simulink model "ProcessFlowRateModel_symbiotic_2014APR18"  (Simulink 7.9)
settings: Solver=VariableStepDiscrete  StartTime=0.0  StopTime=10000  RelTol=1e-3
libraries: simeventslib x9
(part 1 of 2)
settings Model: Creator=tsprock3  LastModifiedBy=tsprock3
settings DebuggingCC: SimStateOlderReleaseMsg=warning

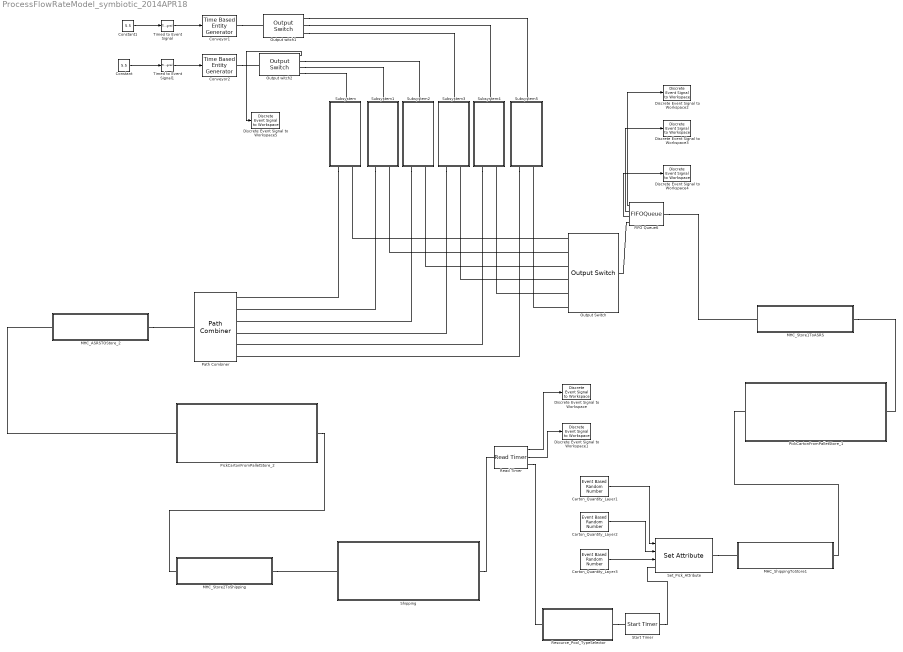
== system ProcessFlowRateModel_symbiotic_2014APR18 ==
  Carton_Quantity_Layer1 : EventBasedRandomNumber  Distribution=Discrete uniform  minUnid=17  maxUnid=23  numValueUnid=7  valueVecDisc=[1 2 3]  probVecDisc=[0.5 0.35 0.15]  Seed=35621
  Carton_Quantity_Layer2 : EventBasedRandomNumber  Distribution=Discrete uniform  minUnid=55  maxUnid=65  numValueUnid=11  valueVecDisc=[1 2 3]  probVecDisc=[0.5 0.35 0.15]  Seed=38838
  Carton_Quantity_Layer3 : EventBasedRandomNumber  Distribution=Discrete uniform  minUnid=17  maxUnid=23  numValueUnid=7  valueVecDisc=[1 2 3]  probVecDisc=[0.5 0.35 0.15]  Seed=42055
  Constant : Constant  Value=5.5
  Constant1 : Constant  Value=5.5
  Conveyor1 : TimeBasedEntityGenerator  GenerateEntitiesUpon=Intergeneration time from port t
  Conveyor2 : TimeBasedEntityGenerator  GenerateEntitiesUpon=Intergeneration time from port t
  Discrete Event Signal to Workspace : simeventslib/SimEvents Sinks/Discrete Event Signal to Workspace  VariableName=elapsedtime  SaveFormat=Structure With Time  isMonitorOnly=off  isRecordIC=off
  Discrete Event Signal to Workspace1 : simeventslib/SimEvents Sinks/Discrete Event Signal to Workspace  VariableName=avg  SaveFormat=Structure With Time  isMonitorOnly=off  isRecordIC=off
  Discrete Event Signal to Workspace2 : simeventslib/SimEvents Sinks/Discrete Event Signal to Workspace  VariableName=serviced_qty  SaveFormat=Structure With Time  isMonitorOnly=off  isRecordIC=off
  Discrete Event Signal to Workspace3 : simeventslib/SimEvents Sinks/Discrete Event Signal to Workspace  VariableName=num_wait  SaveFormat=Structure With Time  isMonitorOnly=off  isRecordIC=off
  Discrete Event Signal to Workspace4 : simeventslib/SimEvents Sinks/Discrete Event Signal to Workspace  VariableName=avg_wait  SaveFormat=Structure With Time  isMonitorOnly=off  isRecordIC=off
  Discrete Event Signal to Workspace5 : simeventslib/SimEvents Sinks/Discrete Event Signal to Workspace  VariableName=intergeneration_time  SaveFormat=Structure With Time  isMonitorOnly=off  isRecordIC=off
  FIFO Queue6 : FIFOQueue  StatNumberDeparted=on  StatNumberInBlock=on  StatAverageWait=on
      settings: OutputPortMap=o0,o1,o2
  MHC_ASRSTOStore_2 : Subsystem
  MHC_ShippingToStore1 : Subsystem
  MHC_Store1ToASRS : Subsystem
  MHC_Store2ToShipping : Subsystem
  Output Switch : OutputSwitch  NumberOutputPorts=6
  Output witch1 : OutputSwitch  SwitchingCriterion=Round robin
  Output witch2 : OutputSwitch  SwitchingCriterion=Round robin  StatNumberDeparted=on
  Path Combiner : PathCombiner  NumberInputPorts=6
  PickCartonFromPalletStore_1 : Subsystem
  PickCartonFromPalletStore_2 : Subsystem
  Read Timer : ReadTimer  StatTimeElapsed=on  StatAverageTimeElapsed=on
      settings: OutputPortMap=o2,o3
  Resource_Pool_TypeSelector : Subsystem  mask{Quantity=24}
      mask prompts: Quantity "How many entities in resource pool?"
  Set_Pick_Attribute : SetAttribute  AttributeName=Carton_Quantity_Layer1|Carton_Quantity_Layer2|Carton_Quantity_Layer3  AttributeFrom=Signal port|Signal port|Signal port  AttributeValue=1|1|1  AttributeTreatAsVector=1|1|1  EvaluatedAttributeValue={[];[];[]}
      settings: InputPortMap=u0,u1,u2
  Shipping : Subsystem
  Start Timer : StartTimer  TimerStartedOption=Restart
  Subsystem : Subsystem  mask{cartonqty=60, popupqty=40}
      mask prompts: cartonqty "Carton_Qty"; popupqty "PopUp_Qty"
  Subsystem1 : Subsystem  mask{cartonqty=60, popupqty=40}
      mask prompts: cartonqty "Carton_Qty"; popupqty "PopUp_Qty"
  Subsystem2 : Subsystem  mask{cartonqty=60, popupqty=40}
      mask prompts: cartonqty "Carton_Qty"; popupqty "PopUp_Qty"
  Subsystem3 : Subsystem  mask{cartonqty=60, popupqty=40}
      mask prompts: cartonqty "Carton_Qty"; popupqty "PopUp_Qty"
  Subsystem4 : Subsystem  mask{cartonqty=60, popupqty=40}
      mask prompts: cartonqty "Carton_Qty"; popupqty "PopUp_Qty"
  Subsystem5 : Subsystem  mask{cartonqty=60, popupqty=40}
      mask prompts: cartonqty "Carton_Qty"; popupqty "PopUp_Qty"
  Timed to Event Signal : TimedToEventSignal
  Timed to Event Signal1 : TimedToEventSignal
  wires:
  Read Timer/1 -> Discrete Event Signal to Workspace/1
  Read Timer/2 -> Discrete Event Signal to Workspace1/1
  Carton_Quantity_Layer1/1 -> Set_Pick_Attribute/1
  Carton_Quantity_Layer2/1 -> Set_Pick_Attribute/2
  Carton_Quantity_Layer3/1 -> Set_Pick_Attribute/3
  FIFO Queue6/3 -> Discrete Event Signal to Workspace4/1
  FIFO Queue6/2 -> Discrete Event Signal to Workspace3/1
  FIFO Queue6/1 -> Discrete Event Signal to Workspace2/1
  Constant1/1 -> Timed to Event Signal/1
  Timed to Event Signal/1 -> Conveyor1/1
  Constant/1 -> Timed to Event Signal1/1
  Timed to Event Signal1/1 -> Conveyor2/1
  Output witch2/1 -> Discrete Event Signal to Workspace5/1
  connections:
  Set_Pick_Attribute/RConn1 -- MHC_ShippingToStore1/LConn1
  MHC_Store2ToShipping/RConn1 -- Shipping/LConn1
  MHC_ShippingToStore1/RConn1 -- PickCartonFromPalletStore_1/LConn1
  MHC_Store1ToASRS/LConn1 -- PickCartonFromPalletStore_1/RConn1
  PickCartonFromPalletStore_2/RConn1 -- MHC_Store2ToShipping/LConn1
  MHC_ASRSTOStore_2/RConn1 -- PickCartonFromPalletStore_2/LConn1
  Conveyor1/RConn1 -- Output witch1/LConn1
  FIFO Queue6/LConn1 -- MHC_Store1ToASRS/RConn1
  Shipping/RConn1 -- Read Timer/LConn1
  Resource_Pool_TypeSelector/LConn1 -- Start Timer/LConn1
  Start Timer/RConn1 -- Set_Pick_Attribute/LConn1
  Read Timer/RConn1 -- Resource_Pool_TypeSelector/RConn1
  MHC_ASRSTOStore_2/LConn1 -- Path Combiner/RConn1
  Output Switch/LConn1 -- FIFO Queue6/RConn1
  Subsystem/RConn1 -- Path Combiner/LConn1
  Conveyor2/RConn1 -- Output witch2/LConn1
  Output witch2/RConn3 -- Subsystem/LConn1
  Output witch2/RConn2 -- Subsystem1/LConn1
  Output witch2/RConn1 -- Subsystem2/LConn1
  Output witch1/RConn3 -- Subsystem3/LConn1
  Output witch1/RConn2 -- Subsystem4/LConn1
  Output witch1/RConn1 -- Subsystem5/LConn1
  Output Switch/RConn1 -- Subsystem/RConn2
  Output Switch/RConn2 -- Subsystem1/RConn2
  Output Switch/RConn3 -- Subsystem2/RConn2
  Output Switch/RConn4 -- Subsystem3/RConn2
  Output Switch/RConn5 -- Subsystem4/RConn2
  Output Switch/RConn6 -- Subsystem5/RConn2
  Subsystem1/RConn1 -- Path Combiner/LConn2
  Subsystem2/RConn1 -- Path Combiner/LConn3
  Subsystem3/RConn1 -- Path Combiner/LConn4
  Subsystem4/RConn1 -- Path Combiner/LConn5
  Subsystem5/RConn1 -- Path Combiner/LConn6

== system ProcessFlowRateModel_symbiotic_2014APR18/MHC_ASRSTOStore_2 ==
  note: This level provides an interface to access the Transportation_Channel block variant. The interface provides a method to
      | bring shipments in and route shipments out, as well as a consistent method to add ports to realize that interface
  IN_Shipment : PathCombiner  NumberInputPorts=1
  OUT_Shipment : OutputSwitch  NumberOutputPorts=1  AttributeName=Customer
  Transportation_Channel : Subsystem
  IN_Shipment_1 : PMIOPort  Port=1  Side=Left
  OUT_Shipment_1 : PMIOPort  Port=2  Side=Right
  connections:
  IN_Shipment/RConn1 -- Transportation_Channel/LConn1
  Transportation_Channel/RConn1 -- OUT_Shipment/LConn1
  IN_Shipment_1/RConn1 -- IN_Shipment/LConn1
  OUT_Shipment/RConn1 -- OUT_Shipment_1/RConn1

== system ProcessFlowRateModel_symbiotic_2014APR18/MHC_ShippingToStore1 ==
  note: This level provides an interface to access the Transportation_Channel block variant. The interface provides a method to
      | bring shipments in and route shipments out, as well as a consistent method to add ports to realize that interface
  IN_Shipment : PathCombiner  NumberInputPorts=1
  OUT_Shipment : OutputSwitch  NumberOutputPorts=1  AttributeName=Customer
  Transportation_Channel : Subsystem
  IN_Shipment_1 : PMIOPort  Port=1  Side=Left
  OUT_Shipment_1 : PMIOPort  Port=2  Side=Right
  connections:
  IN_Shipment/RConn1 -- Transportation_Channel/LConn1
  Transportation_Channel/RConn1 -- OUT_Shipment/LConn1
  IN_Shipment_1/RConn1 -- IN_Shipment/LConn1
  OUT_Shipment/RConn1 -- OUT_Shipment_1/RConn1

== system ProcessFlowRateModel_symbiotic_2014APR18/MHC_Store1ToASRS ==
  note: This level provides an interface to access the Transportation_Channel block variant. The interface provides a method to
      | bring shipments in and route shipments out, as well as a consistent method to add ports to realize that interface
  IN_Shipment : PathCombiner  NumberInputPorts=1
  OUT_Shipment : OutputSwitch  NumberOutputPorts=1  AttributeName=Customer
  Transportation_Channel : Subsystem
  IN_Shipment_1 : PMIOPort  Port=1  Side=Left
  OUT_Shipment_1 : PMIOPort  Port=2  Side=Right
  connections:
  IN_Shipment/RConn1 -- Transportation_Channel/LConn1
  Transportation_Channel/RConn1 -- OUT_Shipment/LConn1
  IN_Shipment_1/RConn1 -- IN_Shipment/LConn1
  OUT_Shipment/RConn1 -- OUT_Shipment_1/RConn1

== system ProcessFlowRateModel_symbiotic_2014APR18/MHC_Store2ToShipping ==
  note: This level provides an interface to access the Transportation_Channel block variant. The interface provides a method to
      | bring shipments in and route shipments out, as well as a consistent method to add ports to realize that interface
  IN_Shipment : PathCombiner  NumberInputPorts=1
  OUT_Shipment : OutputSwitch  NumberOutputPorts=1  AttributeName=Customer
  Transportation_Channel : Subsystem
  IN_Shipment_1 : PMIOPort  Port=1  Side=Left
  OUT_Shipment_1 : PMIOPort  Port=2  Side=Right
  connections:
  IN_Shipment/RConn1 -- Transportation_Channel/LConn1
  Transportation_Channel/RConn1 -- OUT_Shipment/LConn1
  IN_Shipment_1/RConn1 -- IN_Shipment/LConn1
  OUT_Shipment/RConn1 -- OUT_Shipment_1/RConn1

== system ProcessFlowRateModel_symbiotic_2014APR18/PickCartonFromPalletStore_1 ==
  IN_Job : PathCombiner  NumberInputPorts=1
  OUT_Job : OutputSwitch  NumberOutputPorts=1  SwitchingCriterion=Equiprobable  InitialSeed=9514
  Workstation : Subsystem
  IN_Job_1 : PMIOPort  Port=1  Side=Left
  OUT_Job_1 : PMIOPort  Port=2  Side=Right
  connections:
  IN_Job/RConn1 -- Workstation/LConn1
  Workstation/RConn1 -- OUT_Job/LConn1
  IN_Job_1/RConn1 -- IN_Job/LConn1
  OUT_Job/RConn1 -- OUT_Job_1/RConn1

== system ProcessFlowRateModel_symbiotic_2014APR18/PickCartonFromPalletStore_2 ==
  IN_Job : PathCombiner  NumberInputPorts=1
  OUT_Job : OutputSwitch  NumberOutputPorts=1  SwitchingCriterion=Equiprobable  InitialSeed=12731
  Workstation : Subsystem
  IN_Job_1 : PMIOPort  Port=1  Side=Left
  OUT_Job_1 : PMIOPort  Port=2  Side=Right
  connections:
  IN_Job/RConn1 -- Workstation/LConn1
  Workstation/RConn1 -- OUT_Job/LConn1
  IN_Job_1/RConn1 -- IN_Job/LConn1
  OUT_Job/RConn1 -- OUT_Job_1/RConn1

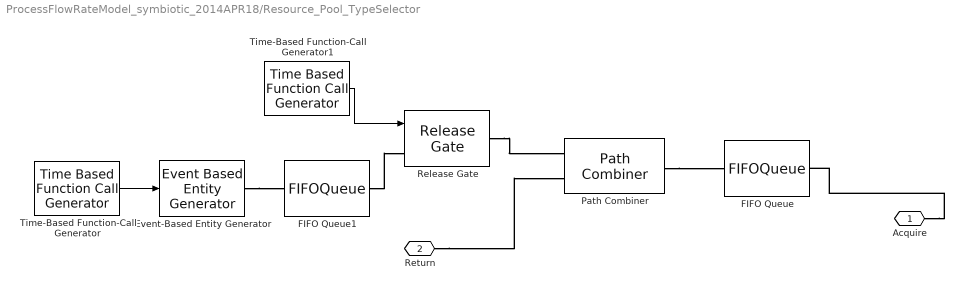
== system ProcessFlowRateModel_symbiotic_2014APR18/Resource_Pool_TypeSelector ==
  Event-Based Entity Generator : EventBasedEntityGenerator  GenerateEntitiesUpon=Function call from port fcn
  FIFO Queue : FIFOQueue  Capacity=inf
  FIFO Queue1 : FIFOQueue  Capacity=inf
  Path Combiner : PathCombiner  NumberInputPorts=2
  Release Gate : ReleaseGate  OpenGateUpon=Function call from port fcn
  Time-Based Function-Call Generator : TimeBasedFunctionCallGenerator  EventGenerationMode=Only at simulation start  NumberOfEventsPerPeriod=Quantity
  Time-Based Function-Call Generator1 : TimeBasedFunctionCallGenerator
  Acquire : PMIOPort  Port=1  Side=Left
  Return : PMIOPort  Port=2  Side=Right
  wires:
  Time-Based Function-Call Generator/1 -> Event-Based Entity Generator/1
  Time-Based Function-Call Generator1/1 -> Release Gate/1
  connections:
  Path Combiner/RConn1 -- FIFO Queue/LConn1
  Return/RConn1 -- Path Combiner/LConn2
  Acquire/RConn1 -- FIFO Queue/RConn1
  Event-Based Entity Generator/RConn1 -- FIFO Queue1/LConn1
  Release Gate/RConn1 -- Path Combiner/LConn1
  FIFO Queue1/RConn1 -- Release Gate/LConn1

== system ProcessFlowRateModel_symbiotic_2014APR18/Shipping ==
  IN_Job : PathCombiner  NumberInputPorts=1
  OUT_Job : OutputSwitch  NumberOutputPorts=1  SwitchingCriterion=Equiprobable  InitialSeed=15948
  Workstation : Subsystem
  IN_Job_1 : PMIOPort  Port=1  Side=Left
  OUT_Job_1 : PMIOPort  Port=2  Side=Right
  connections:
  IN_Job/RConn1 -- Workstation/LConn1
  Workstation/RConn1 -- OUT_Job/LConn1
  IN_Job_1/RConn1 -- IN_Job/LConn1
  OUT_Job/RConn1 -- OUT_Job_1/RConn1

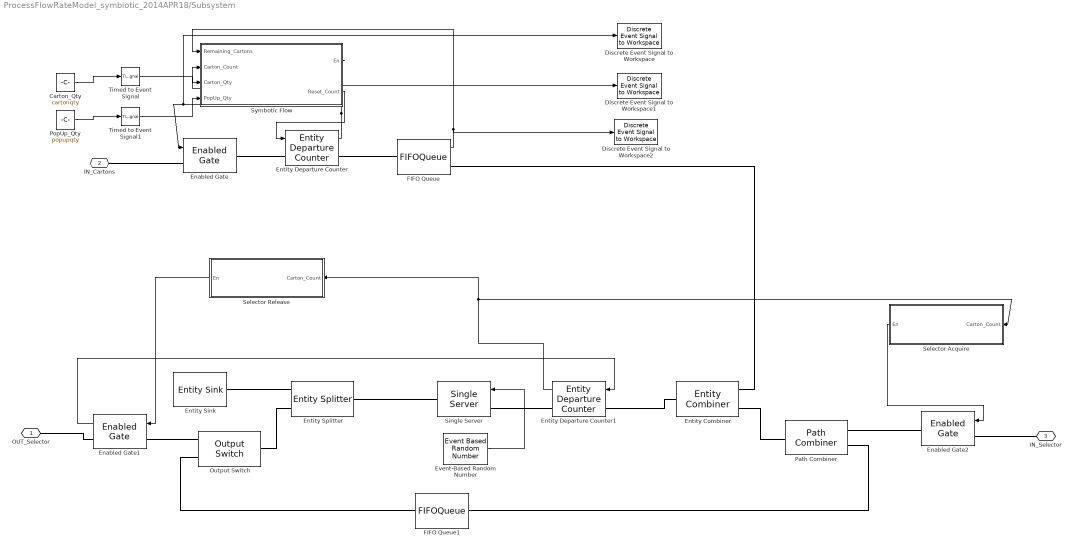
== system ProcessFlowRateModel_symbiotic_2014APR18/Subsystem ==
  Carton_Qty : Constant  Value=cartonqty
  Discrete Event Signal to Workspace : simeventslib/SimEvents Sinks/Discrete Event Signal to Workspace  VariableName=enabled  SaveFormat=Structure With Time  isMonitorOnly=off  isRecordIC=off
  Discrete Event Signal to Workspace1 : simeventslib/SimEvents Sinks/Discrete Event Signal to Workspace  VariableName=pickcount  SaveFormat=Structure With Time  isMonitorOnly=off  isRecordIC=off
  Discrete Event Signal to Workspace2 : simeventslib/SimEvents Sinks/Discrete Event Signal to Workspace  VariableName=accumulatorlength  SaveFormat=Structure With Time  isMonitorOnly=off  isRecordIC=off
  Enabled Gate : EnabledGate
  Enabled Gate1 : EnabledGate  StatNumberDeparted=on
  Enabled Gate2 : EnabledGate
  Entity Combiner : EntityCombiner  NumberInputPorts=2
  Entity Departure Counter : EntityDepartureCounter  NumberDepartedToSignal=on  NumberDepartedToAttribute=off  CounterResetTypeOption=Change in signal from port vc
  Entity Departure Counter1 : EntityDepartureCounter  NumberDepartedToSignal=on  NumberDepartedToAttribute=off  CounterResetTypeOption=Change in signal from port vc
  Entity Sink : EntitySink
  Entity Splitter : EntitySplitter  NumberOutputPorts=2
  Event-Based Random Number : EventBasedRandomNumber  Distribution=Gaussian (normal)  meanNorm=20  stdNorm=5  Seed=13927
  FIFO Queue : FIFOQueue  Capacity=inf  StatNumberInBlock=on
      settings: OutputPortMap=o1
  FIFO Queue1 : FIFOQueue
  Output Switch : OutputSwitch  NumberOutputPorts=2
  Path Combiner : PathCombiner  NumberInputPorts=2
  PopUp_Qty : Constant  Value=popupqty
  Selector Acquire : Truth Table  TreatAsAtomicUnit=on
  Selector Release : Truth Table  TreatAsAtomicUnit=on
  Single Server : SingleServer  ServiceTimeFrom=Signal port t
  Symbotic Flow : Truth Table  TreatAsAtomicUnit=on
  Timed to Event Signal : TimedToEventSignal
  Timed to Event Signal1 : TimedToEventSignal
  OUT_Selector : PMIOPort  Port=1  Side=Right
  IN_Cartons : PMIOPort  Port=2  Side=Left
  IN_Selector : PMIOPort  Port=3  Side=Right
  wires:
  Entity Departure Counter/1 -> Discrete Event Signal to Workspace1/1, Symbotic Flow/2(Carton_Count)
  FIFO Queue/1 -> Discrete Event Signal to Workspace2/1, Symbotic Flow/1(Remaining_Cartons)
  Symbotic Flow/1(En) -> Enabled Gate/1, Discrete Event Signal to Workspace/1
  Event-Based Random Number/1 -> Single Server/1
  Selector Release/1(En) -> Enabled Gate1/1
  Entity Departure Counter1/1 -> Selector Release/1(Carton_Count), Selector Acquire/1(Carton_Count)
  Selector Acquire/1(En) -> Enabled Gate2/1
  Symbotic Flow/2(Reset_Count) -> Entity Departure Counter/1
  Enabled Gate1/1 -> Entity Departure Counter1/1
  Carton_Qty/1 -> Timed to Event Signal/1
  Timed to Event Signal/1 -> Symbotic Flow/3(Carton_Qty)
  PopUp_Qty/1 -> Timed to Event Signal1/1
  Timed to Event Signal1/1 -> Symbotic Flow/4(PopUp_Qty)
  connections:
  Enabled Gate/RConn1 -- Entity Departure Counter/LConn1
  IN_Cartons/RConn1 -- Enabled Gate/LConn1
  Entity Departure Counter/RConn1 -- FIFO Queue/LConn1
  FIFO Queue/RConn1 -- Entity Combiner/LConn1
  Entity Sink/LConn1 -- Entity Splitter/RConn1
  Output Switch/LConn1 -- Entity Splitter/RConn2
  Entity Combiner/LConn2 -- Path Combiner/RConn1
  Enabled Gate1/LConn1 -- Output Switch/RConn1
  OUT_Selector/RConn1 -- Enabled Gate1/RConn1
  Path Combiner/LConn1 -- Enabled Gate2/RConn1
  Enabled Gate2/LConn1 -- IN_Selector/RConn1
  Output Switch/RConn2 -- FIFO Queue1/LConn1
  FIFO Queue1/RConn1 -- Path Combiner/LConn2
  Entity Splitter/LConn1 -- Single Server/RConn1
  Single Server/LConn1 -- Entity Departure Counter1/RConn1
  Entity Departure Counter1/LConn1 -- Entity Combiner/RConn1

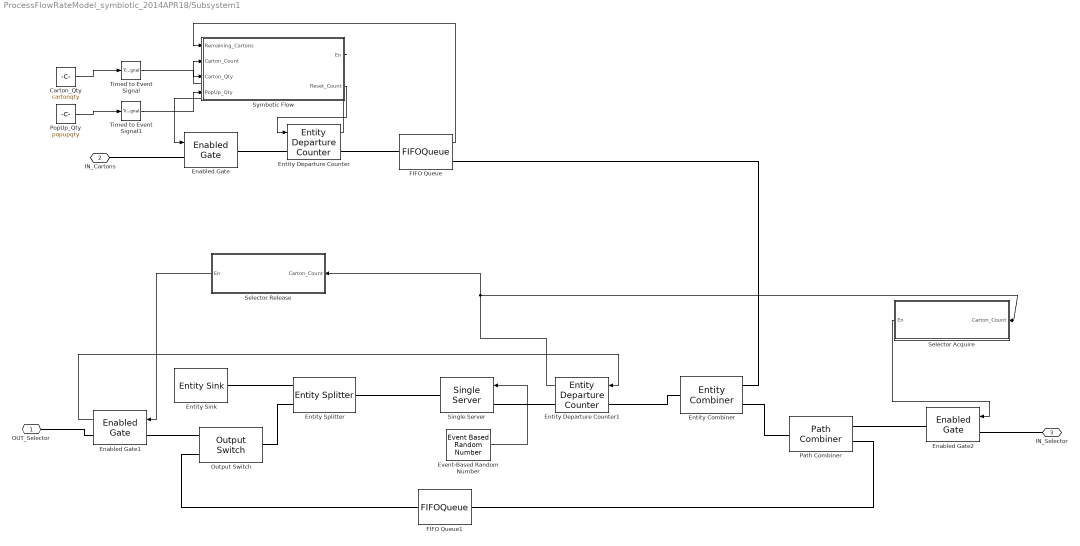
== system ProcessFlowRateModel_symbiotic_2014APR18/Subsystem1 ==
  Carton_Qty : Constant  Value=cartonqty
  Enabled Gate : EnabledGate
  Enabled Gate1 : EnabledGate  StatNumberDeparted=on
  Enabled Gate2 : EnabledGate
  Entity Combiner : EntityCombiner  NumberInputPorts=2
  Entity Departure Counter : EntityDepartureCounter  NumberDepartedToSignal=on  NumberDepartedToAttribute=off  CounterResetTypeOption=Change in signal from port vc
  Entity Departure Counter1 : EntityDepartureCounter  NumberDepartedToSignal=on  NumberDepartedToAttribute=off  CounterResetTypeOption=Change in signal from port vc
  Entity Sink : EntitySink
  Entity Splitter : EntitySplitter  NumberOutputPorts=2
  Event-Based Random Number : EventBasedRandomNumber  Distribution=Gaussian (normal)  meanNorm=20  stdNorm=5  Seed=17144
  FIFO Queue : FIFOQueue  Capacity=inf  StatNumberInBlock=on
      settings: OutputPortMap=o1
  FIFO Queue1 : FIFOQueue
  Output Switch : OutputSwitch  NumberOutputPorts=2
  Path Combiner : PathCombiner  NumberInputPorts=2
  PopUp_Qty : Constant  Value=popupqty
  Selector Acquire : Truth Table  TreatAsAtomicUnit=on
  Selector Release : Truth Table  TreatAsAtomicUnit=on
  Single Server : SingleServer  ServiceTimeFrom=Signal port t
  Symbotic Flow : Truth Table  TreatAsAtomicUnit=on
  Timed to Event Signal : TimedToEventSignal
  Timed to Event Signal1 : TimedToEventSignal
  OUT_Selector : PMIOPort  Port=1  Side=Right
  IN_Cartons : PMIOPort  Port=2  Side=Left
  IN_Selector : PMIOPort  Port=3  Side=Right
  wires:
  Entity Departure Counter/1 -> Symbotic Flow/2(Carton_Count)
  FIFO Queue/1 -> Symbotic Flow/1(Remaining_Cartons)
  Symbotic Flow/1(En) -> Enabled Gate/1
  Event-Based Random Number/1 -> Single Server/1
  Selector Release/1(En) -> Enabled Gate1/1
  Entity Departure Counter1/1 -> Selector Release/1(Carton_Count), Selector Acquire/1(Carton_Count)
  Selector Acquire/1(En) -> Enabled Gate2/1
  Symbotic Flow/2(Reset_Count) -> Entity Departure Counter/1
  Enabled Gate1/1 -> Entity Departure Counter1/1
  Carton_Qty/1 -> Timed to Event Signal/1
  Timed to Event Signal/1 -> Symbotic Flow/3(Carton_Qty)
  PopUp_Qty/1 -> Timed to Event Signal1/1
  Timed to Event Signal1/1 -> Symbotic Flow/4(PopUp_Qty)
  connections:
  Enabled Gate/RConn1 -- Entity Departure Counter/LConn1
  IN_Cartons/RConn1 -- Enabled Gate/LConn1
  Entity Departure Counter/RConn1 -- FIFO Queue/LConn1
  FIFO Queue/RConn1 -- Entity Combiner/LConn1
  Entity Sink/LConn1 -- Entity Splitter/RConn1
  Output Switch/LConn1 -- Entity Splitter/RConn2
  Entity Combiner/LConn2 -- Path Combiner/RConn1
  Enabled Gate1/LConn1 -- Output Switch/RConn1
  OUT_Selector/RConn1 -- Enabled Gate1/RConn1
  Path Combiner/LConn1 -- Enabled Gate2/RConn1
  Enabled Gate2/LConn1 -- IN_Selector/RConn1
  Output Switch/RConn2 -- FIFO Queue1/LConn1
  FIFO Queue1/RConn1 -- Path Combiner/LConn2
  Entity Splitter/LConn1 -- Single Server/RConn1
  Single Server/LConn1 -- Entity Departure Counter1/RConn1
  Entity Departure Counter1/LConn1 -- Entity Combiner/RConn1

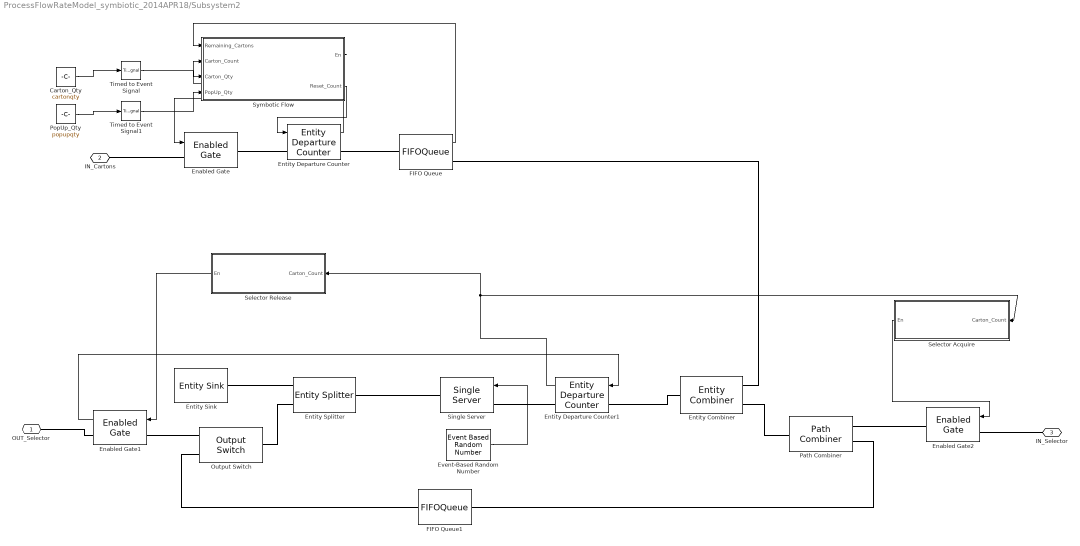
== system ProcessFlowRateModel_symbiotic_2014APR18/Subsystem2 ==
  Carton_Qty : Constant  Value=cartonqty
  Enabled Gate : EnabledGate
  Enabled Gate1 : EnabledGate  StatNumberDeparted=on
  Enabled Gate2 : EnabledGate
  Entity Combiner : EntityCombiner  NumberInputPorts=2
  Entity Departure Counter : EntityDepartureCounter  NumberDepartedToSignal=on  NumberDepartedToAttribute=off  CounterResetTypeOption=Change in signal from port vc
  Entity Departure Counter1 : EntityDepartureCounter  NumberDepartedToSignal=on  NumberDepartedToAttribute=off  CounterResetTypeOption=Change in signal from port vc
  Entity Sink : EntitySink
  Entity Splitter : EntitySplitter  NumberOutputPorts=2
  Event-Based Random Number : EventBasedRandomNumber  Distribution=Gaussian (normal)  meanNorm=20  stdNorm=5  Seed=20361
  FIFO Queue : FIFOQueue  Capacity=inf  StatNumberInBlock=on
      settings: OutputPortMap=o1
  FIFO Queue1 : FIFOQueue
  Output Switch : OutputSwitch  NumberOutputPorts=2
  Path Combiner : PathCombiner  NumberInputPorts=2
  PopUp_Qty : Constant  Value=popupqty
  Selector Acquire : Truth Table  TreatAsAtomicUnit=on
  Selector Release : Truth Table  TreatAsAtomicUnit=on
  Single Server : SingleServer  ServiceTimeFrom=Signal port t
  Symbotic Flow : Truth Table  TreatAsAtomicUnit=on
  Timed to Event Signal : TimedToEventSignal
  Timed to Event Signal1 : TimedToEventSignal
  OUT_Selector : PMIOPort  Port=1  Side=Right
  IN_Cartons : PMIOPort  Port=2  Side=Left
  IN_Selector : PMIOPort  Port=3  Side=Right
  wires:
  Entity Departure Counter/1 -> Symbotic Flow/2(Carton_Count)
  FIFO Queue/1 -> Symbotic Flow/1(Remaining_Cartons)
  Symbotic Flow/1(En) -> Enabled Gate/1
  Event-Based Random Number/1 -> Single Server/1
  Selector Release/1(En) -> Enabled Gate1/1
  Entity Departure Counter1/1 -> Selector Release/1(Carton_Count), Selector Acquire/1(Carton_Count)
  Selector Acquire/1(En) -> Enabled Gate2/1
  Symbotic Flow/2(Reset_Count) -> Entity Departure Counter/1
  Enabled Gate1/1 -> Entity Departure Counter1/1
  Carton_Qty/1 -> Timed to Event Signal/1
  Timed to Event Signal/1 -> Symbotic Flow/3(Carton_Qty)
  PopUp_Qty/1 -> Timed to Event Signal1/1
  Timed to Event Signal1/1 -> Symbotic Flow/4(PopUp_Qty)
  connections:
  Enabled Gate/RConn1 -- Entity Departure Counter/LConn1
  IN_Cartons/RConn1 -- Enabled Gate/LConn1
  Entity Departure Counter/RConn1 -- FIFO Queue/LConn1
  FIFO Queue/RConn1 -- Entity Combiner/LConn1
  Entity Sink/LConn1 -- Entity Splitter/RConn1
  Output Switch/LConn1 -- Entity Splitter/RConn2
  Entity Combiner/LConn2 -- Path Combiner/RConn1
  Enabled Gate1/LConn1 -- Output Switch/RConn1
  OUT_Selector/RConn1 -- Enabled Gate1/RConn1
  Path Combiner/LConn1 -- Enabled Gate2/RConn1
  Enabled Gate2/LConn1 -- IN_Selector/RConn1
  Output Switch/RConn2 -- FIFO Queue1/LConn1
  FIFO Queue1/RConn1 -- Path Combiner/LConn2
  Entity Splitter/LConn1 -- Single Server/RConn1
  Single Server/LConn1 -- Entity Departure Counter1/RConn1
  Entity Departure Counter1/LConn1 -- Entity Combiner/RConn1

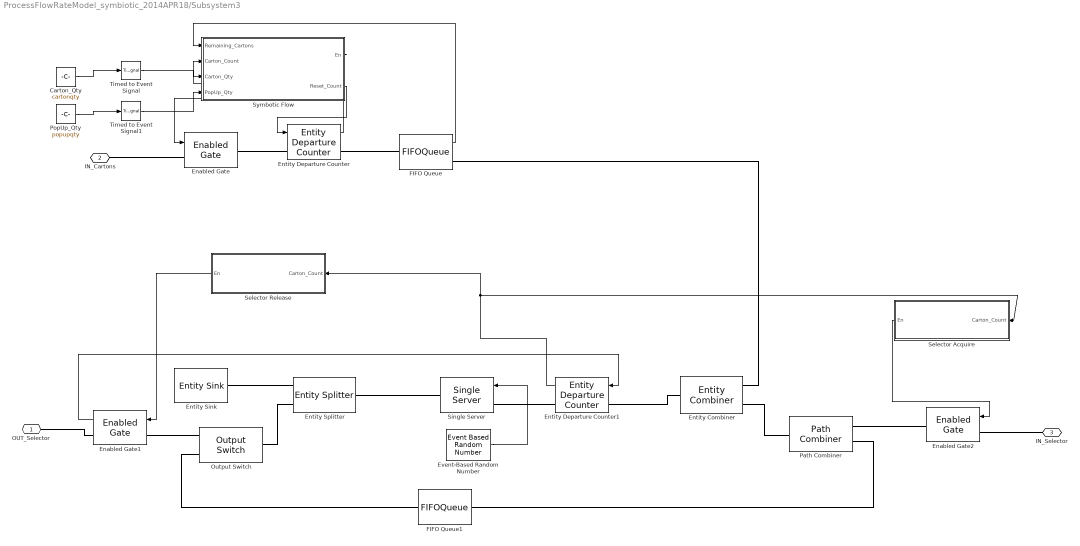
== system ProcessFlowRateModel_symbiotic_2014APR18/Subsystem3 ==
  Carton_Qty : Constant  Value=cartonqty
  Enabled Gate : EnabledGate
  Enabled Gate1 : EnabledGate  StatNumberDeparted=on
  Enabled Gate2 : EnabledGate
  Entity Combiner : EntityCombiner  NumberInputPorts=2
  Entity Departure Counter : EntityDepartureCounter  NumberDepartedToSignal=on  NumberDepartedToAttribute=off  CounterResetTypeOption=Change in signal from port vc
  Entity Departure Counter1 : EntityDepartureCounter  NumberDepartedToSignal=on  NumberDepartedToAttribute=off  CounterResetTypeOption=Change in signal from port vc
  Entity Sink : EntitySink
  Entity Splitter : EntitySplitter  NumberOutputPorts=2
  Event-Based Random Number : EventBasedRandomNumber  Distribution=Gaussian (normal)  meanNorm=20  stdNorm=5  Seed=26795
  FIFO Queue : FIFOQueue  Capacity=inf  StatNumberInBlock=on
      settings: OutputPortMap=o1
  FIFO Queue1 : FIFOQueue
  Output Switch : OutputSwitch  NumberOutputPorts=2
  Path Combiner : PathCombiner  NumberInputPorts=2
  PopUp_Qty : Constant  Value=popupqty
  Selector Acquire : Truth Table  TreatAsAtomicUnit=on
  Selector Release : Truth Table  TreatAsAtomicUnit=on
  Single Server : SingleServer  ServiceTimeFrom=Signal port t
  Symbotic Flow : Truth Table  TreatAsAtomicUnit=on
  Timed to Event Signal : TimedToEventSignal
  Timed to Event Signal1 : TimedToEventSignal
  OUT_Selector : PMIOPort  Port=1  Side=Right
  IN_Cartons : PMIOPort  Port=2  Side=Left
  IN_Selector : PMIOPort  Port=3  Side=Right
  wires:
  Entity Departure Counter/1 -> Symbotic Flow/2(Carton_Count)
  FIFO Queue/1 -> Symbotic Flow/1(Remaining_Cartons)
  Symbotic Flow/1(En) -> Enabled Gate/1
  Event-Based Random Number/1 -> Single Server/1
  Selector Release/1(En) -> Enabled Gate1/1
  Entity Departure Counter1/1 -> Selector Release/1(Carton_Count), Selector Acquire/1(Carton_Count)
  Selector Acquire/1(En) -> Enabled Gate2/1
  Symbotic Flow/2(Reset_Count) -> Entity Departure Counter/1
  Enabled Gate1/1 -> Entity Departure Counter1/1
  Carton_Qty/1 -> Timed to Event Signal/1
  Timed to Event Signal/1 -> Symbotic Flow/3(Carton_Qty)
  PopUp_Qty/1 -> Timed to Event Signal1/1
  Timed to Event Signal1/1 -> Symbotic Flow/4(PopUp_Qty)
  connections:
  Enabled Gate/RConn1 -- Entity Departure Counter/LConn1
  IN_Cartons/RConn1 -- Enabled Gate/LConn1
  Entity Departure Counter/RConn1 -- FIFO Queue/LConn1
  FIFO Queue/RConn1 -- Entity Combiner/LConn1
  Entity Sink/LConn1 -- Entity Splitter/RConn1
  Output Switch/LConn1 -- Entity Splitter/RConn2
  Entity Combiner/LConn2 -- Path Combiner/RConn1
  Enabled Gate1/LConn1 -- Output Switch/RConn1
  OUT_Selector/RConn1 -- Enabled Gate1/RConn1
  Path Combiner/LConn1 -- Enabled Gate2/RConn1
  Enabled Gate2/LConn1 -- IN_Selector/RConn1
  Output Switch/RConn2 -- FIFO Queue1/LConn1
  FIFO Queue1/RConn1 -- Path Combiner/LConn2
  Entity Splitter/LConn1 -- Single Server/RConn1
  Single Server/LConn1 -- Entity Departure Counter1/RConn1
  Entity Departure Counter1/LConn1 -- Entity Combiner/RConn1

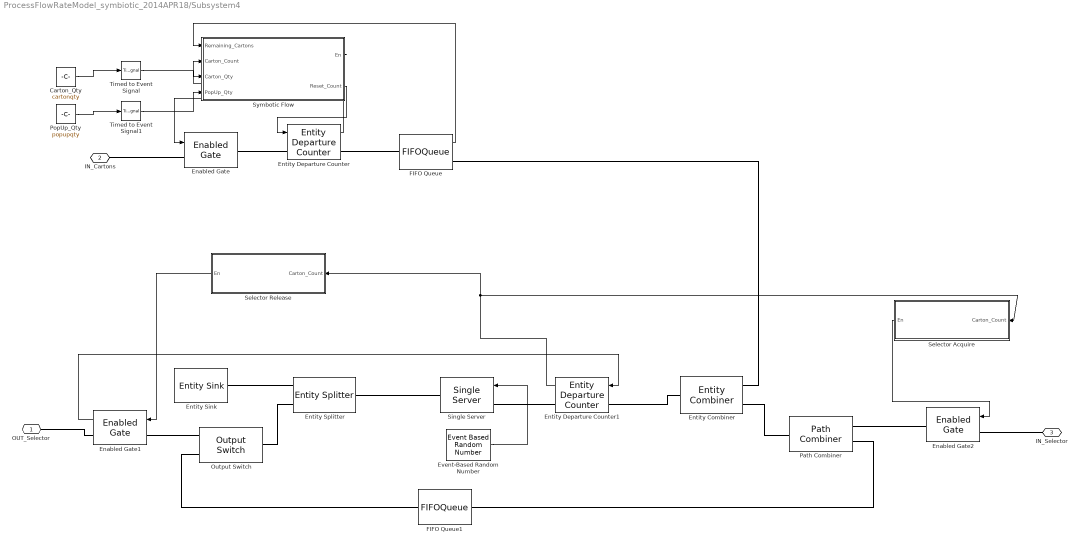
== system ProcessFlowRateModel_symbiotic_2014APR18/Subsystem4 ==
  Carton_Qty : Constant  Value=cartonqty
  Enabled Gate : EnabledGate
  Enabled Gate1 : EnabledGate  StatNumberDeparted=on
  Enabled Gate2 : EnabledGate
  Entity Combiner : EntityCombiner  NumberInputPorts=2
  Entity Departure Counter : EntityDepartureCounter  NumberDepartedToSignal=on  NumberDepartedToAttribute=off  CounterResetTypeOption=Change in signal from port vc
  Entity Departure Counter1 : EntityDepartureCounter  NumberDepartedToSignal=on  NumberDepartedToAttribute=off  CounterResetTypeOption=Change in signal from port vc
  Entity Sink : EntitySink
  Entity Splitter : EntitySplitter  NumberOutputPorts=2
  Event-Based Random Number : EventBasedRandomNumber  Distribution=Gaussian (normal)  meanNorm=20  stdNorm=5  Seed=30012
  FIFO Queue : FIFOQueue  Capacity=inf  StatNumberInBlock=on
      settings: OutputPortMap=o1
  FIFO Queue1 : FIFOQueue
  Output Switch : OutputSwitch  NumberOutputPorts=2
  Path Combiner : PathCombiner  NumberInputPorts=2
  PopUp_Qty : Constant  Value=popupqty
  Selector Acquire : Truth Table  TreatAsAtomicUnit=on
  Selector Release : Truth Table  TreatAsAtomicUnit=on
  Single Server : SingleServer  ServiceTimeFrom=Signal port t
  Symbotic Flow : Truth Table  TreatAsAtomicUnit=on
  Timed to Event Signal : TimedToEventSignal
  Timed to Event Signal1 : TimedToEventSignal
  OUT_Selector : PMIOPort  Port=1  Side=Right
  IN_Cartons : PMIOPort  Port=2  Side=Left
  IN_Selector : PMIOPort  Port=3  Side=Right
  wires:
  Entity Departure Counter/1 -> Symbotic Flow/2(Carton_Count)
  FIFO Queue/1 -> Symbotic Flow/1(Remaining_Cartons)
  Symbotic Flow/1(En) -> Enabled Gate/1
  Event-Based Random Number/1 -> Single Server/1
  Selector Release/1(En) -> Enabled Gate1/1
  Entity Departure Counter1/1 -> Selector Release/1(Carton_Count), Selector Acquire/1(Carton_Count)
  Selector Acquire/1(En) -> Enabled Gate2/1
  Symbotic Flow/2(Reset_Count) -> Entity Departure Counter/1
  Enabled Gate1/1 -> Entity Departure Counter1/1
  Carton_Qty/1 -> Timed to Event Signal/1
  Timed to Event Signal/1 -> Symbotic Flow/3(Carton_Qty)
  PopUp_Qty/1 -> Timed to Event Signal1/1
  Timed to Event Signal1/1 -> Symbotic Flow/4(PopUp_Qty)
  connections:
  Enabled Gate/RConn1 -- Entity Departure Counter/LConn1
  IN_Cartons/RConn1 -- Enabled Gate/LConn1
  Entity Departure Counter/RConn1 -- FIFO Queue/LConn1
  FIFO Queue/RConn1 -- Entity Combiner/LConn1
  Entity Sink/LConn1 -- Entity Splitter/RConn1
  Output Switch/LConn1 -- Entity Splitter/RConn2
  Entity Combiner/LConn2 -- Path Combiner/RConn1
  Enabled Gate1/LConn1 -- Output Switch/RConn1
  OUT_Selector/RConn1 -- Enabled Gate1/RConn1
  Path Combiner/LConn1 -- Enabled Gate2/RConn1
  Enabled Gate2/LConn1 -- IN_Selector/RConn1
  Output Switch/RConn2 -- FIFO Queue1/LConn1
  FIFO Queue1/RConn1 -- Path Combiner/LConn2
  Entity Splitter/LConn1 -- Single Server/RConn1
  Single Server/LConn1 -- Entity Departure Counter1/RConn1
  Entity Departure Counter1/LConn1 -- Entity Combiner/RConn1

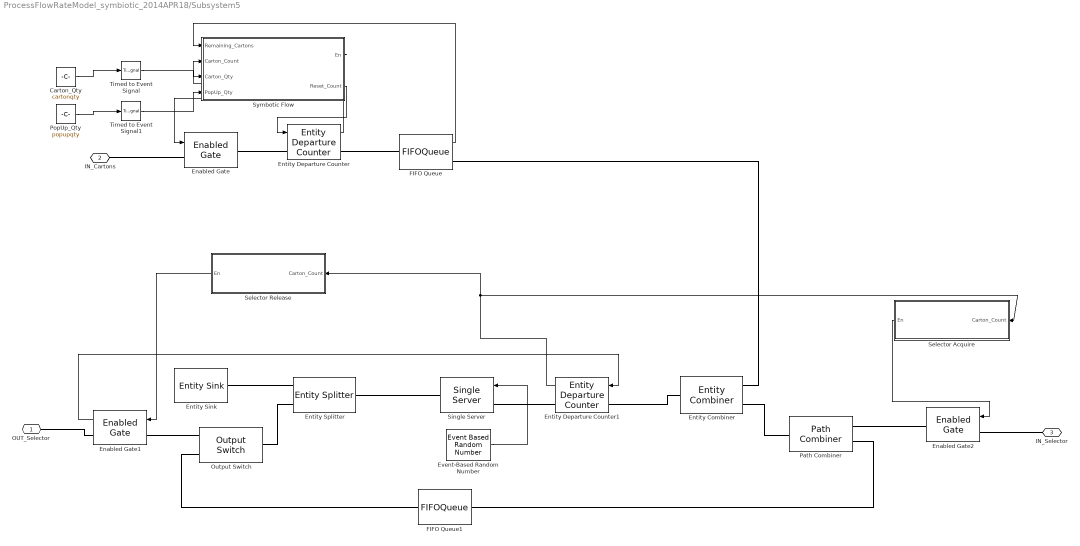
== system ProcessFlowRateModel_symbiotic_2014APR18/Subsystem5 ==
  Carton_Qty : Constant  Value=cartonqty
  Enabled Gate : EnabledGate
  Enabled Gate1 : EnabledGate  StatNumberDeparted=on
  Enabled Gate2 : EnabledGate
  Entity Combiner : EntityCombiner  NumberInputPorts=2
  Entity Departure Counter : EntityDepartureCounter  NumberDepartedToSignal=on  NumberDepartedToAttribute=off  CounterResetTypeOption=Change in signal from port vc
  Entity Departure Counter1 : EntityDepartureCounter  NumberDepartedToSignal=on  NumberDepartedToAttribute=off  CounterResetTypeOption=Change in signal from port vc
  Entity Sink : EntitySink
  Entity Splitter : EntitySplitter  NumberOutputPorts=2
  Event-Based Random Number : EventBasedRandomNumber  Distribution=Gaussian (normal)  meanNorm=20  stdNorm=5  Seed=33229
  FIFO Queue : FIFOQueue  Capacity=inf  StatNumberInBlock=on
      settings: OutputPortMap=o1
  FIFO Queue1 : FIFOQueue
  Output Switch : OutputSwitch  NumberOutputPorts=2
  Path Combiner : PathCombiner  NumberInputPorts=2
  PopUp_Qty : Constant  Value=popupqty
  Selector Acquire : Truth Table  TreatAsAtomicUnit=on
  Selector Release : Truth Table  TreatAsAtomicUnit=on
  Single Server : SingleServer  ServiceTimeFrom=Signal port t
  Symbotic Flow : Truth Table  TreatAsAtomicUnit=on
  Timed to Event Signal : TimedToEventSignal
  Timed to Event Signal1 : TimedToEventSignal
  OUT_Selector : PMIOPort  Port=1  Side=Right
  IN_Cartons : PMIOPort  Port=2  Side=Left
  IN_Selector : PMIOPort  Port=3  Side=Right
  wires:
  Entity Departure Counter/1 -> Symbotic Flow/2(Carton_Count)
  FIFO Queue/1 -> Symbotic Flow/1(Remaining_Cartons)
  Symbotic Flow/1(En) -> Enabled Gate/1
  Event-Based Random Number/1 -> Single Server/1
  Selector Release/1(En) -> Enabled Gate1/1
  Entity Departure Counter1/1 -> Selector Release/1(Carton_Count), Selector Acquire/1(Carton_Count)
  Selector Acquire/1(En) -> Enabled Gate2/1
  Symbotic Flow/2(Reset_Count) -> Entity Departure Counter/1
  Enabled Gate1/1 -> Entity Departure Counter1/1
  Carton_Qty/1 -> Timed to Event Signal/1
  Timed to Event Signal/1 -> Symbotic Flow/3(Carton_Qty)
  PopUp_Qty/1 -> Timed to Event Signal1/1
  Timed to Event Signal1/1 -> Symbotic Flow/4(PopUp_Qty)
  connections:
  Enabled Gate/RConn1 -- Entity Departure Counter/LConn1
  IN_Cartons/RConn1 -- Enabled Gate/LConn1
  Entity Departure Counter/RConn1 -- FIFO Queue/LConn1
  FIFO Queue/RConn1 -- Entity Combiner/LConn1
  Entity Sink/LConn1 -- Entity Splitter/RConn1
  Output Switch/LConn1 -- Entity Splitter/RConn2
  Entity Combiner/LConn2 -- Path Combiner/RConn1
  Enabled Gate1/LConn1 -- Output Switch/RConn1
  OUT_Selector/RConn1 -- Enabled Gate1/RConn1
  Path Combiner/LConn1 -- Enabled Gate2/RConn1
  Enabled Gate2/LConn1 -- IN_Selector/RConn1
  Output Switch/RConn2 -- FIFO Queue1/LConn1
  FIFO Queue1/RConn1 -- Path Combiner/LConn2
  Entity Splitter/LConn1 -- Single Server/RConn1
  Single Server/LConn1 -- Entity Departure Counter1/RConn1
  Entity Departure Counter1/LConn1 -- Entity Combiner/RConn1

== system ProcessFlowRateModel_symbiotic_2014APR18/MHC_ASRSTOStore_2/Transportation_Channel ==
  FIFO Queue : FIFOQueue  Capacity=inf
  N-Server : NServer  NumberOfServers=inf  ServiceTime=10
  IN_Shipment : PMIOPort  Port=1  Side=Left
  OUT_Shipment : PMIOPort  Port=2  Side=Right
  connections:
  FIFO Queue/RConn1 -- N-Server/LConn1
  IN_Shipment/RConn1 -- FIFO Queue/LConn1
  OUT_Shipment/RConn1 -- N-Server/RConn1

== system ProcessFlowRateModel_symbiotic_2014APR18/MHC_ShippingToStore1/Transportation_Channel ==
  FIFO Queue : FIFOQueue  Capacity=inf
  N-Server : NServer  NumberOfServers=inf  ServiceTime=20
  IN_Shipment : PMIOPort  Port=1  Side=Left
  OUT_Shipment : PMIOPort  Port=2  Side=Right
  connections:
  FIFO Queue/RConn1 -- N-Server/LConn1
  IN_Shipment/RConn1 -- FIFO Queue/LConn1
  OUT_Shipment/RConn1 -- N-Server/RConn1

== system ProcessFlowRateModel_symbiotic_2014APR18/MHC_Store1ToASRS/Transportation_Channel ==
  FIFO Queue : FIFOQueue  Capacity=inf
  N-Server : NServer  NumberOfServers=inf  ServiceTime=10
  IN_Shipment : PMIOPort  Port=1  Side=Left
  OUT_Shipment : PMIOPort  Port=2  Side=Right
  connections:
  FIFO Queue/RConn1 -- N-Server/LConn1
  IN_Shipment/RConn1 -- FIFO Queue/LConn1
  OUT_Shipment/RConn1 -- N-Server/RConn1

== system ProcessFlowRateModel_symbiotic_2014APR18/MHC_Store2ToShipping/Transportation_Channel ==
  FIFO Queue : FIFOQueue  Capacity=inf
  N-Server : NServer  NumberOfServers=inf  ServiceTime=20
  IN_Shipment : PMIOPort  Port=1  Side=Left
  OUT_Shipment : PMIOPort  Port=2  Side=Right
  connections:
  FIFO Queue/RConn1 -- N-Server/LConn1
  IN_Shipment/RConn1 -- FIFO Queue/LConn1
  OUT_Shipment/RConn1 -- N-Server/RConn1

== system ProcessFlowRateModel_symbiotic_2014APR18/PickCartonFromPalletStore_1/Workstation ==
  CartonPick : Subsystem
  Entity_Combiner : EntityCombiner  NumberInputPorts=1
  Entity_Splitter : EntitySplitter  NumberOutputPorts=1
  FIFO Queue : FIFOQueue
  OUT_Job_1 : PMIOPort  Port=1  Side=Right
  IN_Job_1 : PMIOPort  Port=2  Side=Left
  connections:
  FIFO Queue/RConn1 -- Entity_Combiner/LConn1
  Entity_Splitter/RConn1 -- OUT_Job_1/RConn1
  IN_Job_1/RConn1 -- FIFO Queue/LConn1
  Entity_Combiner/RConn1 -- CartonPick/LConn1
  CartonPick/RConn1 -- Entity_Splitter/LConn1

== system ProcessFlowRateModel_symbiotic_2014APR18/PickCartonFromPalletStore_2/Workstation ==
  CartonPick : Subsystem
  Entity_Combiner : EntityCombiner  NumberInputPorts=1
  Entity_Splitter : EntitySplitter  NumberOutputPorts=1
  FIFO Queue : FIFOQueue
  OUT_Job_1 : PMIOPort  Port=1  Side=Right
  IN_Job_1 : PMIOPort  Port=2  Side=Left
  connections:
  FIFO Queue/RConn1 -- Entity_Combiner/LConn1
  Entity_Splitter/RConn1 -- OUT_Job_1/RConn1
  IN_Job_1/RConn1 -- FIFO Queue/LConn1
  Entity_Combiner/RConn1 -- CartonPick/LConn1
  CartonPick/RConn1 -- Entity_Splitter/LConn1

== system ProcessFlowRateModel_symbiotic_2014APR18/Shipping/Workstation ==
  Entity_Combiner : EntityCombiner  NumberInputPorts=1
  Entity_Splitter : EntitySplitter  NumberOutputPorts=1
  FIFO Queue : FIFOQueue
  Shipping : Subsystem
  OUT_Job_1 : PMIOPort  Port=1  Side=Right
  IN_Job_1 : PMIOPort  Port=2  Side=Left
  connections:
  FIFO Queue/RConn1 -- Entity_Combiner/LConn1
  Entity_Splitter/RConn1 -- OUT_Job_1/RConn1
  IN_Job_1/RConn1 -- FIFO Queue/LConn1
  Entity_Combiner/RConn1 -- Shipping/LConn1
  Shipping/RConn1 -- Entity_Splitter/LConn1

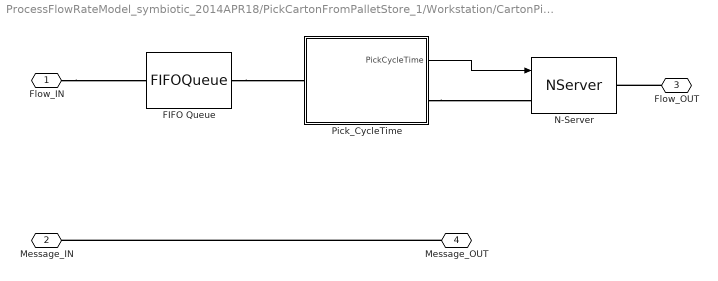
== system ProcessFlowRateModel_symbiotic_2014APR18/PickCartonFromPalletStore_1/Workstation/CartonPick ==
  FIFO Queue : FIFOQueue
  N-Server : NServer  NumberOfServers=inf  ServiceTimeFrom=Signal port t  ServiceTime=0
  Pick_CycleTime : Subsystem  mask{pickmean=5, pickstddev=0.25, traveltime=80}
      mask prompts: pickmean "eachPickMean"; pickstddev "eachPickStdDev"
  Flow_IN : PMIOPort  Port=1  Side=Left
  Message_IN : PMIOPort  Port=2  Side=Left
  Flow_OUT : PMIOPort  Port=3  Side=Right
  Message_OUT : PMIOPort  Port=4  Side=Right
  wires:
  Pick_CycleTime/1(PickCycleTime) -> N-Server/1
  connections:
  Flow_IN/RConn1 -- FIFO Queue/LConn1
  Flow_OUT/RConn1 -- N-Server/RConn1
  Message_OUT/RConn1 -- Message_IN/RConn1
  FIFO Queue/RConn1 -- Pick_CycleTime/LConn1
  Pick_CycleTime/RConn1 -- N-Server/LConn1

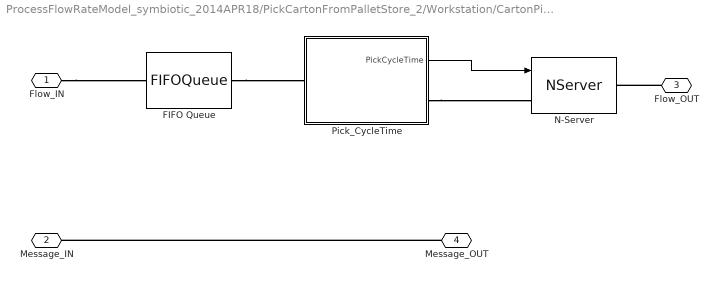
== system ProcessFlowRateModel_symbiotic_2014APR18/PickCartonFromPalletStore_2/Workstation/CartonPick ==
  FIFO Queue : FIFOQueue
  N-Server : NServer  NumberOfServers=inf  ServiceTimeFrom=Signal port t  ServiceTime=0
  Pick_CycleTime : Subsystem  mask{pickmean=5, pickstddev=0.25, traveltime=80}
      mask prompts: pickmean "eachPickMean"; pickstddev "eachPickStdDev"
  Flow_IN : PMIOPort  Port=1  Side=Left
  Message_IN : PMIOPort  Port=2  Side=Left
  Flow_OUT : PMIOPort  Port=3  Side=Right
  Message_OUT : PMIOPort  Port=4  Side=Right
  wires:
  Pick_CycleTime/1(PickCycleTime) -> N-Server/1
  connections:
  Flow_IN/RConn1 -- FIFO Queue/LConn1
  Flow_OUT/RConn1 -- N-Server/RConn1
  Message_OUT/RConn1 -- Message_IN/RConn1
  FIFO Queue/RConn1 -- Pick_CycleTime/LConn1
  Pick_CycleTime/RConn1 -- N-Server/LConn1

== system ProcessFlowRateModel_symbiotic_2014APR18/Shipping/Workstation/Shipping ==
  IN_Job : PathCombiner  NumberInputPorts=1
  OUT_Job : OutputSwitch  NumberOutputPorts=1  SwitchingCriterion=Equiprobable  InitialSeed=65399
  Process : Subsystem
  IN_Job_1 : PMIOPort  Port=1  Side=Left
  OUT_Job_1 : PMIOPort  Port=2  Side=Right
  connections:
  IN_Job/RConn1 -- Process/LConn1
  Process/RConn1 -- OUT_Job/LConn1
  IN_Job_1/RConn1 -- IN_Job/LConn1
  OUT_Job_1/RConn1 -- OUT_Job/RConn1

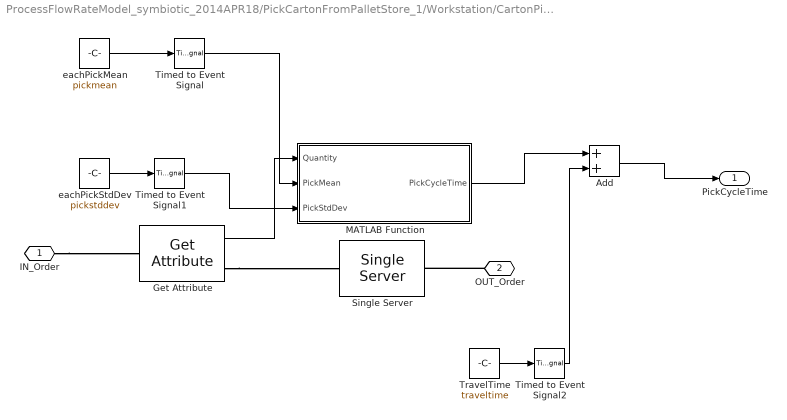
== system ProcessFlowRateModel_symbiotic_2014APR18/PickCartonFromPalletStore_1/Workstation/CartonPick/Pick_CycleTime ==
  Add : Sum
  Get Attribute : GetAttribute  AttributeName=Carton_Quantity_Layer1  EvaluatedDefaultAttributeValue={[]}
      settings: OutputPortMap=o1
  MATLAB Function : MATLAB Function  TreatAsAtomicUnit=on
  Single Server : SingleServer  ServiceTime=0
  Timed to Event Signal : TimedToEventSignal
  Timed to Event Signal1 : TimedToEventSignal
  Timed to Event Signal2 : TimedToEventSignal
  TravelTime : Constant  Value=traveltime
  eachPickMean : Constant  Value=pickmean
  eachPickStdDev : Constant  Value=pickstddev
  IN_Order : PMIOPort  Port=1  Side=Left
  OUT_Order : PMIOPort  Port=2  Side=Right
  PickCycleTime : Outport
  wires:
  Get Attribute/1 -> MATLAB Function/1(Quantity)
  MATLAB Function/1(PickCycleTime) -> Add/1
  Add/1 -> PickCycleTime/1
  eachPickStdDev/1 -> Timed to Event Signal1/1
  Timed to Event Signal1/1 -> MATLAB Function/3(PickStdDev)
  eachPickMean/1 -> Timed to Event Signal/1
  Timed to Event Signal/1 -> MATLAB Function/2(PickMean)
  TravelTime/1 -> Timed to Event Signal2/1
  Timed to Event Signal2/1 -> Add/2
  connections:
  Get Attribute/RConn1 -- Single Server/LConn1
  IN_Order/RConn1 -- Get Attribute/LConn1
  OUT_Order/RConn1 -- Single Server/RConn1

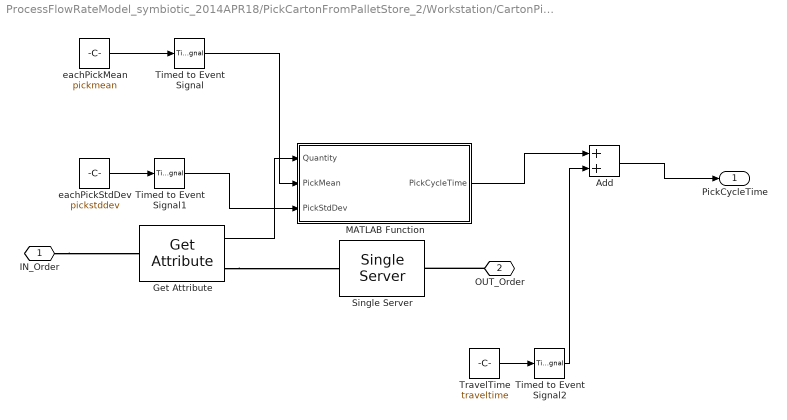
== system ProcessFlowRateModel_symbiotic_2014APR18/PickCartonFromPalletStore_2/Workstation/CartonPick/Pick_CycleTime ==
  Add : Sum
  Get Attribute : GetAttribute  AttributeName=Carton_Quantity_Layer3  EvaluatedDefaultAttributeValue={[]}
      settings: OutputPortMap=o1
  MATLAB Function : MATLAB Function  TreatAsAtomicUnit=on
  Single Server : SingleServer  ServiceTime=0
  Timed to Event Signal : TimedToEventSignal
  Timed to Event Signal1 : TimedToEventSignal
  Timed to Event Signal2 : TimedToEventSignal
  TravelTime : Constant  Value=traveltime
  eachPickMean : Constant  Value=pickmean
  eachPickStdDev : Constant  Value=pickstddev
  IN_Order : PMIOPort  Port=1  Side=Left
  OUT_Order : PMIOPort  Port=2  Side=Right
  PickCycleTime : Outport
  wires:
  Get Attribute/1 -> MATLAB Function/1(Quantity)
  MATLAB Function/1(PickCycleTime) -> Add/1
  Add/1 -> PickCycleTime/1
  eachPickStdDev/1 -> Timed to Event Signal1/1
  Timed to Event Signal1/1 -> MATLAB Function/3(PickStdDev)
  eachPickMean/1 -> Timed to Event Signal/1
  Timed to Event Signal/1 -> MATLAB Function/2(PickMean)
  TravelTime/1 -> Timed to Event Signal2/1
  Timed to Event Signal2/1 -> Add/2
  connections:
  Get Attribute/RConn1 -- Single Server/LConn1
  IN_Order/RConn1 -- Get Attribute/LConn1
  OUT_Order/RConn1 -- Single Server/RConn1

== system ProcessFlowRateModel_symbiotic_2014APR18/Shipping/Workstation/Shipping/Process ==
  FIFO Queue : FIFOQueue  Capacity=inf
  N-Server : NServer  NumberOfServers=inf  ServiceTimeFrom=Signal port t
  ProcessTime : EventBasedRandomNumber  Distribution=Arbitrary discrete  minUnif=1  meanNorm=5  minUnid=29.9  maxUnid=30  numValueUnid=1  valueVecDisc=[0 30]  probVecDisc=[0 1]  Seed=58965
  Job_OUT : PMIOPort  Port=1  Side=Right
  Job_IN : PMIOPort  Port=2  Side=Left
  wires:
  ProcessTime/1 -> N-Server/1
  connections:
  FIFO Queue/RConn1 -- N-Server/LConn1
  Job_OUT/RConn1 -- N-Server/RConn1
  Job_IN/RConn1 -- FIFO Queue/LConn1

== matlab function PickCartonFromPalletStore_2/Workstation/CartonPick/Pick_CycleTime/MATLAB Function ==
  data: Quantity input double; PickCycleTime output double; PickMean input double; PickStdDev input double
function PickCycleTime = fcn(Quantity,  PickMean, PickStdDev)
%#codegen

coder.extrinsic('normrnd');
PickCycleTime = zeros(1, 'double');

Pick_Mean = Quantity*PickMean;
Pick_StdDev =Quantity*PickStdDev;

PickCycleTime = normrnd(Pick_Mean, sqrt(Pick_StdDev));

== matlab function Subsystem/Symbotic Flow ==
  data: Remaining_Cartons input double; En output double; Carton_Count input double; Reset_Count output double; Carton_Qty input double; PopUp_Qty input double
function [En, Reset_Count] = fcn(Remaining_Cartons, Carton_Count, Carton_Qty, PopUp_Qty)

aVarTruthTableCondition_1 = false;
aVarTruthTableCondition_2 = false;


% Order fully picked

aVarTruthTableCondition_1 = logical(Carton_Count == (Carton_Qty-1));

% Accumulator Available

aVarTruthTableCondition_2 = logical(Remaining_Cartons <= PopUp_Qty);

if (aVarTruthTableCondition_1 && aVarTruthTableCondition_2)
    aFcnTruthTableAction_1();
elseif (aVarTruthTableCondition_1 && ~aVarTruthTableCondition_2)
    aFcnTruthTableAction_2();
elseif (~aVarTruthTableCondition_1 && aVarTruthTableCondition_2)
    aFcnTruthTableAction_3();
else % Default
    aFcnTruthTableAction_3();
end

function aFcnTruthTableAction_1()

% Allow accumulator flow
% reset count

En = 1;
Reset_Count = 1;

function aFcnTruthTableAction_2()

% Halt accumulator flow
% Do not reset

En = 0;
Reset_Count = 0;

function aFcnTruthTableAction_3()

% Allow accumulator flow
% Do not reset

En = 1;
Reset_Count = 0;

== matlab function Subsystem/Selector Release ==
  data: En output double; Carton_Count input double
function En = fcn(Carton_Count)

aVarTruthTableCondition_1 = false;


% Order fully picked

aVarTruthTableCondition_1 = logical(Carton_Count == 60);

if (aVarTruthTableCondition_1)
    aFcnTruthTableAction_1();
else % Default
    aFcnTruthTableAction_2();
end

function aFcnTruthTableAction_1()

% Release Selector

En = 1;

function aFcnTruthTableAction_2()

% Return Selector

En = 0;

== matlab function Subsystem/Selector Acquire ==
  data: En output double; Carton_Count input double
function En = fcn(Carton_Count)

aVarTruthTableCondition_1 = false;


% New Order

aVarTruthTableCondition_1 = logical(Carton_Count == 0);

if (aVarTruthTableCondition_1)
    aFcnTruthTableAction_1();
else % Default
    aFcnTruthTableAction_2();
end

function aFcnTruthTableAction_1()

% Release Selector

En = 1;

function aFcnTruthTableAction_2()

% Return Selector

En = 0;

== matlab function Subsystem1/Selector Acquire ==
  data: En output double; Carton_Count input double
function En = fcn(Carton_Count)

aVarTruthTableCondition_1 = false;


% New Order

aVarTruthTableCondition_1 = logical(Carton_Count == 0);

if (aVarTruthTableCondition_1)
    aFcnTruthTableAction_1();
else % Default
    aFcnTruthTableAction_2();
end

function aFcnTruthTableAction_1()

% Release Selector

En = 1;

function aFcnTruthTableAction_2()

% Return Selector

En = 0;

== matlab function Subsystem1/Selector Release ==
  data: En output double; Carton_Count input double
function En = fcn(Carton_Count)

aVarTruthTableCondition_1 = false;


% Order fully picked

aVarTruthTableCondition_1 = logical(Carton_Count == 60);

if (aVarTruthTableCondition_1)
    aFcnTruthTableAction_1();
else % Default
    aFcnTruthTableAction_2();
end

function aFcnTruthTableAction_1()

% Release Selector

En = 1;

function aFcnTruthTableAction_2()

% Return Selector

En = 0;

== matlab function Subsystem1/Symbotic Flow ==
  data: Remaining_Cartons input double; En output double; Carton_Count input double; Reset_Count output double; Carton_Qty input double; PopUp_Qty input double
function [En, Reset_Count] = fcn(Remaining_Cartons, Carton_Count, Carton_Qty, PopUp_Qty)

aVarTruthTableCondition_1 = false;
aVarTruthTableCondition_2 = false;


% Order fully picked

aVarTruthTableCondition_1 = logical(Carton_Count == (Carton_Qty-1));

% Accumulator Available

aVarTruthTableCondition_2 = logical(Remaining_Cartons <= PopUp_Qty);

if (aVarTruthTableCondition_1 && aVarTruthTableCondition_2)
    aFcnTruthTableAction_1();
elseif (aVarTruthTableCondition_1 && ~aVarTruthTableCondition_2)
    aFcnTruthTableAction_2();
elseif (~aVarTruthTableCondition_1 && aVarTruthTableCondition_2)
    aFcnTruthTableAction_3();
else % Default
    aFcnTruthTableAction_3();
end

function aFcnTruthTableAction_1()

% Allow accumulator flow
% reset count

En = 1;
Reset_Count = 1;

function aFcnTruthTableAction_2()

% Halt accumulator flow
% Do not reset

En = 0;
Reset_Count = 0;

function aFcnTruthTableAction_3()

% Allow accumulator flow
% Do not reset

En = 1;
Reset_Count = 0;

== matlab function Subsystem2/Selector Acquire ==
  data: En output double; Carton_Count input double
function En = fcn(Carton_Count)

aVarTruthTableCondition_1 = false;


% New Order

aVarTruthTableCondition_1 = logical(Carton_Count == 0);

if (aVarTruthTableCondition_1)
    aFcnTruthTableAction_1();
else % Default
    aFcnTruthTableAction_2();
end

function aFcnTruthTableAction_1()

% Release Selector

En = 1;

function aFcnTruthTableAction_2()

% Return Selector

En = 0;

== matlab function Subsystem2/Selector Release ==
  data: En output double; Carton_Count input double
function En = fcn(Carton_Count)

aVarTruthTableCondition_1 = false;


% Order fully picked

aVarTruthTableCondition_1 = logical(Carton_Count == 60);

if (aVarTruthTableCondition_1)
    aFcnTruthTableAction_1();
else % Default
    aFcnTruthTableAction_2();
end

function aFcnTruthTableAction_1()

% Release Selector

En = 1;

function aFcnTruthTableAction_2()

% Return Selector

En = 0;

== matlab function Subsystem2/Symbotic Flow ==
  data: Remaining_Cartons input double; En output double; Carton_Count input double; Reset_Count output double; Carton_Qty input double; PopUp_Qty input double
function [En, Reset_Count] = fcn(Remaining_Cartons, Carton_Count, Carton_Qty, PopUp_Qty)

aVarTruthTableCondition_1 = false;
aVarTruthTableCondition_2 = false;


% Order fully picked

aVarTruthTableCondition_1 = logical(Carton_Count == (Carton_Qty-1));

% Accumulator Available

aVarTruthTableCondition_2 = logical(Remaining_Cartons <= PopUp_Qty);

if (aVarTruthTableCondition_1 && aVarTruthTableCondition_2)
    aFcnTruthTableAction_1();
elseif (aVarTruthTableCondition_1 && ~aVarTruthTableCondition_2)
    aFcnTruthTableAction_2();
elseif (~aVarTruthTableCondition_1 && aVarTruthTableCondition_2)
    aFcnTruthTableAction_3();
else % Default
    aFcnTruthTableAction_3();
end

function aFcnTruthTableAction_1()

% Allow accumulator flow
% reset count

En = 1;
Reset_Count = 1;

function aFcnTruthTableAction_2()

% Halt accumulator flow
% Do not reset

En = 0;
Reset_Count = 0;

function aFcnTruthTableAction_3()

% Allow accumulator flow
% Do not reset

En = 1;
Reset_Count = 0;

== matlab function PickCartonFromPalletStore_1/Workstation/CartonPick/Pick_CycleTime/MATLAB Function ==
  data: Quantity input double; PickCycleTime output double; PickMean input double; PickStdDev input double
function PickCycleTime = fcn(Quantity,  PickMean, PickStdDev)
%#codegen

coder.extrinsic('normrnd');
PickCycleTime = zeros(1, 'double');

Pick_Mean = Quantity*PickMean;
Pick_StdDev =Quantity*PickStdDev;

PickCycleTime = normrnd(Pick_Mean, sqrt(Pick_StdDev));

== matlab function Subsystem3/Selector Acquire ==
  data: En output double; Carton_Count input double
function En = fcn(Carton_Count)

aVarTruthTableCondition_1 = false;


% New Order

aVarTruthTableCondition_1 = logical(Carton_Count == 0);

if (aVarTruthTableCondition_1)
    aFcnTruthTableAction_1();
else % Default
    aFcnTruthTableAction_2();
end

function aFcnTruthTableAction_1()

% Release Selector

En = 1;

function aFcnTruthTableAction_2()

% Return Selector

En = 0;

== matlab function Subsystem3/Selector Release ==
  data: En output double; Carton_Count input double
function En = fcn(Carton_Count)

aVarTruthTableCondition_1 = false;


% Order fully picked

aVarTruthTableCondition_1 = logical(Carton_Count == 60);

if (aVarTruthTableCondition_1)
    aFcnTruthTableAction_1();
else % Default
    aFcnTruthTableAction_2();
end

function aFcnTruthTableAction_1()

% Release Selector

En = 1;

function aFcnTruthTableAction_2()

% Return Selector

En = 0;

== matlab function Subsystem3/Symbotic Flow ==
  data: Remaining_Cartons input double; En output double; Carton_Count input double; Reset_Count output double; Carton_Qty input double; PopUp_Qty input double
function [En, Reset_Count] = fcn(Remaining_Cartons, Carton_Count, Carton_Qty, PopUp_Qty)

aVarTruthTableCondition_1 = false;
aVarTruthTableCondition_2 = false;


% Order fully picked

aVarTruthTableCondition_1 = logical(Carton_Count == (Carton_Qty-1));

% Accumulator Available

aVarTruthTableCondition_2 = logical(Remaining_Cartons <= PopUp_Qty);

if (aVarTruthTableCondition_1 && aVarTruthTableCondition_2)
    aFcnTruthTableAction_1();
elseif (aVarTruthTableCondition_1 && ~aVarTruthTableCondition_2)
    aFcnTruthTableAction_2();
elseif (~aVarTruthTableCondition_1 && aVarTruthTableCondition_2)
    aFcnTruthTableAction_3();
else % Default
    aFcnTruthTableAction_3();
end

function aFcnTruthTableAction_1()

% Allow accumulator flow
% reset count

En = 1;
Reset_Count = 1;

function aFcnTruthTableAction_2()

% Halt accumulator flow
% Do not reset

En = 0;
Reset_Count = 0;

function aFcnTruthTableAction_3()

% Allow accumulator flow
% Do not reset

En = 1;
Reset_Count = 0;
